simulink model "PanelModel"  (R2018a)
settings: Solver=VariableStepAuto  StartTime=0.0  StopTime=10.0  RelTol=1e-3
undefined symbols (not defined in the file): J, Kd
settings Model: Creator=Choaib ELMADI  LastModifiedBy=Choaib ELMADI

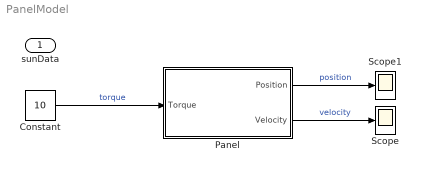
== system PanelModel ==
  sunData : Inport
  Constant : Constant  Value=10
  Panel : Subsystem
  Scope : Scope
  Scope1 : Scope
  wires:
  Constant/1 -> Panel/1(Torque)  "torque"
  Panel/1(Position) -> Scope1/1  "position"
  Panel/2(Velocity) -> Scope/1  "velocity"

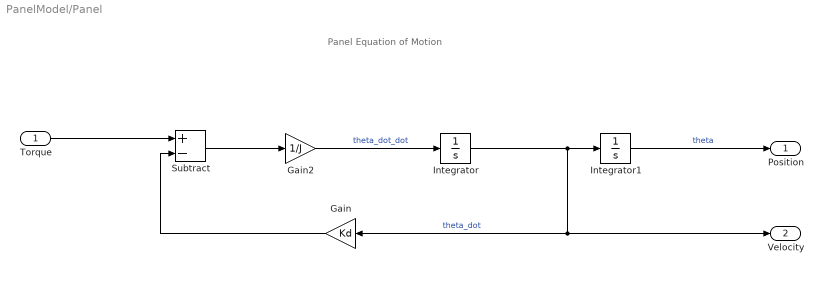
== system PanelModel/Panel ==
  note: Panel Equation of Motion
  Torque : Inport
  Gain : Gain  Gain=Kd
  Gain2 : Gain  Gain=1/J
  Integrator : Integrator
  Integrator1 : Integrator
  Subtract : Sum  Inputs=+-
  Position : Outport
  Velocity : Outport  Port=2
  wires:
  Integrator/1 -> Velocity/1, Gain/1, Integrator1/1  "theta_dot"
  Integrator1/1 -> Position/1  "theta"
  Gain2/1 -> Integrator/1  "theta_dot_dot"
  Torque/1 -> Subtract/1
  Gain/1 -> Subtract/2
  Subtract/1 -> Gain2/1
